simulink model "HOYAS_GRANDES_I"  (R2023b)
settings: Solver=FixedStepDiscrete  StartTime=0.0  StopTime=inf  FixedStep=Ts_Power  RelTol=1e-3  EnableMultiTasking=on
PostLoadFcn:
  | Ts_Power=50e-6;f=50;R_ac=0.12;L_ac=0.08/(2*pi*50);L1=0.17874;L2=0.07596;L3=0.04321;L4=0.01471;L5=0.04751;L6=0.2054;L7=0.17263;L8=0.14418;L9=0.17697;L10=0.19944;L11=0.18905;L12=0.26987;L13=0.1671;L14=0.16874;L15=0.14664;L16=0.12477;L17=0.14989;L18=0.17217;L19=0.19436; load('PV_prof_norm.mat');
InitFcn:
  | Ts_Power=50e-6;f=50;R_ac=0.12;L_ac=0.08/(2*pi*50);L1=0.17874;L2=0.07596;L3=0.04321;L4=0.01471;L5=0.04751;L6=0.2054;L7=0.17263;L8=0.14418;L9=0.17697;L10=0.19944;L11=0.18905;L12=0.26987;L13=0.1671;L14=0.16874;L15=0.14664;L16=0.12477;L17=0.14989;L18=0.17217;L19=0.19436; load('PV_prof_norm.mat');
undefined symbols (not defined in the file or in its folder): D11, Delta, L, X_ac
libraries: spsVoltageMeasurementLib x84, spsCurrentMeasurementLib x75, rtlab x41, spsThreePhaseSeriesRLCBranchLib x38, spsGroundLib x28, powerlib_extras x25, spsThreePhaseDynamicLoadLib x19, eeGeneralControl x4, rteventslib x4, spsThreePhasePISectionLineLib x2, spsThreePhaseTransformerTwoWindingsLib x2, spsPLLLib x1
(part 2 of 4)

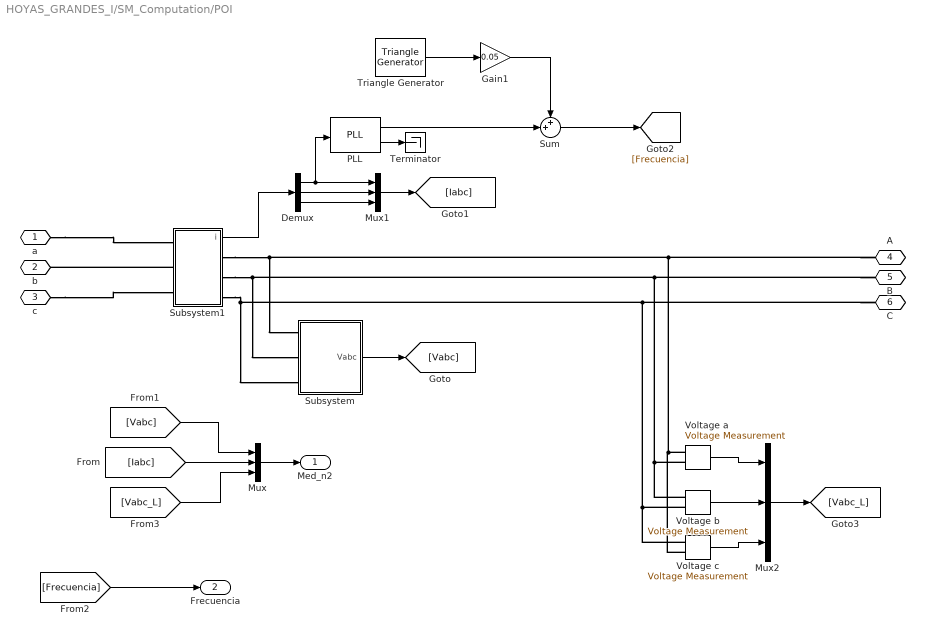
== system HOYAS_GRANDES_I/SM_Computation/POI ==
  Demux : Demux  Outputs=3
  Gain1 : Gain  Gain=0.05
  Mux : Mux  Inputs=3
  Mux1 : Mux  Inputs=3
  Mux2 : Mux  Inputs=3
  PLL : spsPLLLib/PLL  Fmin=45  Par_Init=[0, 50]  ParK=[180, 3200, 1]  TcD=1e-4  MaxRateChangeFreq=12  FilterCutOffFreq=25  Ts=Ts_Power  AGC=on
      settings: LibrarySourceBlock=sps_lib/Control/PLL
  Subsystem : Subsystem
  Subsystem1 : Subsystem
  Sum : Sum  Inputs=++|
  Terminator : Terminator
  Triangle Generator : spsTriangleGeneratorLib/Triangle Generator  Freq=0.1  Phase=0  Ts=Ts_Power
  Voltage a : spsVoltageMeasurementLib/Voltage Measurement  PhasorSimulation=off  OutputType=Complex  PSBequivalent=0
  Voltage b : spsVoltageMeasurementLib/Voltage Measurement  PhasorSimulation=off  OutputType=Complex  PSBequivalent=0
  Voltage c : spsVoltageMeasurementLib/Voltage Measurement  PhasorSimulation=off  OutputType=Complex  PSBequivalent=0
  a : PMIOPort  Side=Right
  b : PMIOPort  Port=2  Side=Right
  c : PMIOPort  Port=3  Side=Right
  A : PMIOPort  Port=4  Side=Left
  B : PMIOPort  Port=5  Side=Left
  C : PMIOPort  Port=6  Side=Left
  Med_n2 : Outport
  Frecuencia : Outport  Port=2
  wires:
  Mux/1 -> Med_n2/1
  [Iabc] -> Mux/2
  [Vabc] -> Mux/1
  Subsystem/1(Vabc) -> [Vabc]
  Mux1/1 -> [Iabc]
  Subsystem1/1(i) -> Demux/1
  Demux/1 -> PLL/1, Mux1/1
  Demux/2 -> Mux1/2
  Demux/3 -> Mux1/3
  PLL/2 -> Terminator/1
  [Frecuencia] -> Frecuencia/1
  Sum/1 -> [Frecuencia]
  Triangle Generator/1 -> Gain1/1
  PLL/1 -> Sum/2
  Gain1/1 -> Sum/1
  Voltage a/1 -> Mux2/1
  Voltage b/1 -> Mux2/2
  Voltage c/1 -> Mux2/3
  Mux2/1 -> [Vabc_L]
  [Vabc_L] -> Mux/3
  connections:
  a/RConn1 -- Subsystem1/LConn1
  Subsystem1/LConn2 -- b/RConn1
  c/RConn1 -- Subsystem1/LConn3
  Voltage c/LConn1 -- Subsystem/LConn3 -- Subsystem1/RConn3 -- C/RConn1 -- Voltage b/LConn2
  Voltage a/LConn1 -- Subsystem/LConn1 -- Subsystem1/RConn1 -- A/RConn1 -- Voltage c/LConn2
  Voltage b/LConn1 -- Subsystem/LConn2 -- Subsystem1/RConn2 -- B/RConn1 -- Voltage a/LConn2

== system HOYAS_GRANDES_I/SM_Computation/Subsystem1 ==
  P_profile : Inport
  P_PPC : Inport  Port=2
  PPC : Constant  Commented=on  Value=0
  Perfil : Constant  Commented=on  Value=3e3
  RTE Conversion : rteventslib/Signal Attributes/RTE Conversion  inputdatatype=RTE Boolean  outputdatatype=Double  compensation=Enabled  nbMaxEvents=10  sampleTime=Ts_Power
      settings: SourceProductName=RT-EVENTS
  RTE Relational Operator1 : rteventslib/Math Operations/RTE Relational Operator  RelationalOperator=>  NumberMaxEvents=1  SampleTime=Ts_Power
      settings: SourceProductName=RT-EVENTS
  Switch : Switch  Criteria=u2 > Threshold  SaturateOnIntegerOverflow=off  InputSameDT=off
  Out1 : Outport
  wires:
  P_profile/1 -> [Perfil]
  P_PPC/1 -> [PPC]
  RTE Relational Operator1/1 -> RTE Conversion/1
  RTE Conversion/1 -> Switch/2
  Switch/1 -> Out1/1
  [Perfil] -> Switch/3, RTE Relational Operator1/1
  [PPC] -> Switch/1, RTE Relational Operator1/2

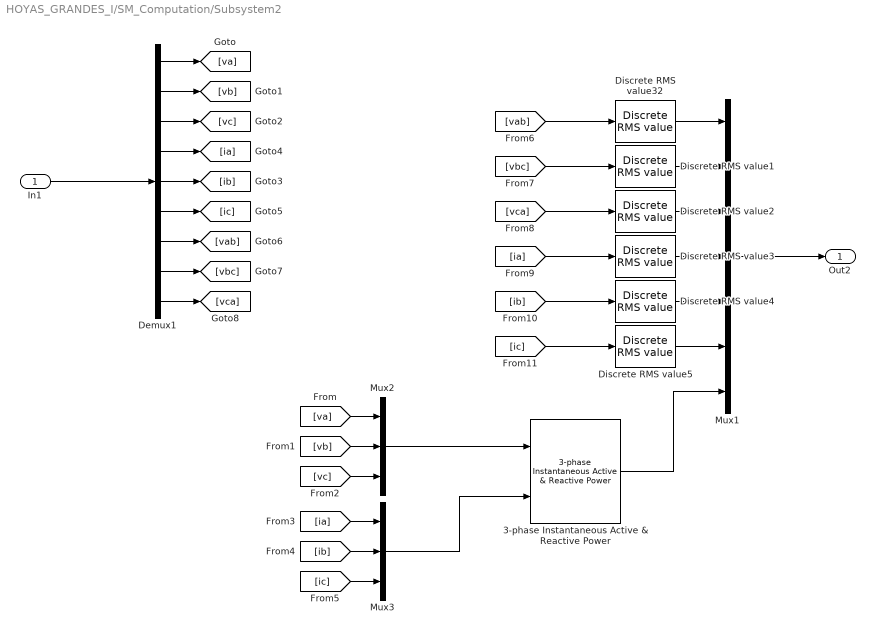
== system HOYAS_GRANDES_I/SM_Computation/Subsystem2 ==
  In1 : Inport
  3-phase Instantaneous Active & Reactive Power : powerlib_extras/Measurements/3-phase  Instantaneous  Active & Reactive Power
  Demux1 : Demux  Outputs=9
  Discrete RMS value1 : powerlib_extras/Discrete Measurements/Discrete  RMS value  Freq=50  Mag_Init=20e3  Ts=Ts_Power
  Discrete RMS value2 : powerlib_extras/Discrete Measurements/Discrete  RMS value  Freq=50  Mag_Init=20e3  Ts=Ts_Power
  Discrete RMS value3 : powerlib_extras/Discrete Measurements/Discrete  RMS value  Freq=50  Mag_Init=0  Ts=Ts_Power
  Discrete RMS value32 : powerlib_extras/Discrete Measurements/Discrete  RMS value  Freq=50  Mag_Init=20e3  Ts=Ts_Power
  Discrete RMS value4 : powerlib_extras/Discrete Measurements/Discrete  RMS value  Freq=50  Mag_Init=0  Ts=Ts_Power
  Discrete RMS value5 : powerlib_extras/Discrete Measurements/Discrete  RMS value  Freq=50  Mag_Init=0  Ts=Ts_Power
  Mux1 : Mux  Inputs=7
  Mux2 : Mux  Inputs=3
  Mux3 : Mux  Inputs=3
  Out2 : Outport
  wires:
  Discrete RMS value5/1 -> Mux1/6
  Discrete RMS value4/1 -> Mux1/5
  Discrete RMS value3/1 -> Mux1/4
  [ic] -> Discrete RMS value5/1
  [ib] -> Discrete RMS value4/1
  [ia] -> Discrete RMS value3/1
  3-phase Instantaneous Active & Reactive Power/1 -> Mux1/7
  [vca] -> Discrete RMS value2/1
  Discrete RMS value2/1 -> Mux1/3
  [vbc] -> Discrete RMS value1/1
  [vab] -> Discrete RMS value32/1
  Demux1/9 -> [vca]
  Demux1/8 -> [vbc]
  Demux1/7 -> [vab]
  [ic] -> Mux3/3
  [ib] -> Mux3/2
  [ia] -> Mux3/1
  [vc] -> Mux2/3
  [vb] -> Mux2/2
  [va] -> Mux2/1
  Mux3/1 -> 3-phase Instantaneous Active & Reactive Power/2
  Mux2/1 -> 3-phase Instantaneous Active & Reactive Power/1
  Demux1/6 -> [ic]
  Demux1/5 -> [ib]
  Demux1/3 -> [vc]
  Demux1/2 -> [vb]
  In1/1 -> Demux1/1
  Demux1/1 -> [va]
  Demux1/4 -> [ia]
  Mux1/1 -> Out2/1
  Discrete RMS value32/1 -> Mux1/1
  Discrete RMS value1/1 -> Mux1/2

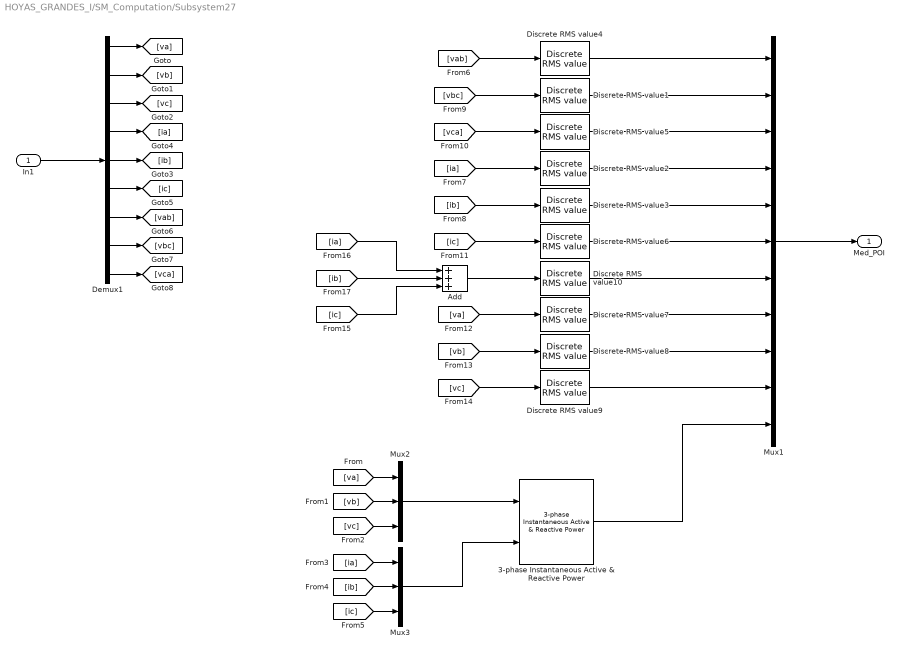
== system HOYAS_GRANDES_I/SM_Computation/Subsystem27 ==
  In1 : Inport
  3-phase Instantaneous Active & Reactive Power : powerlib_extras/Measurements/3-phase  Instantaneous  Active & Reactive Power
  Add : Sum  Inputs=+++
  Demux1 : Demux  Outputs=9
  Discrete RMS value1 : powerlib_extras/Discrete Measurements/Discrete  RMS value  Freq=50  Mag_Init=20e3  Ts=Ts_Power
  Discrete RMS value{2..3,6,10} (4 alike) : powerlib_extras/Discrete Measurements/Discrete  RMS value  Freq=50  Mag_Init=0  Ts=Ts_Power
  Discrete RMS value4 : powerlib_extras/Discrete Measurements/Discrete  RMS value  Freq=50  Mag_Init=20e3  Ts=Ts_Power
  Discrete RMS value5 : powerlib_extras/Discrete Measurements/Discrete  RMS value  Freq=50  Mag_Init=20e3  Ts=Ts_Power
  Discrete RMS value7 : powerlib_extras/Discrete Measurements/Discrete  RMS value  Freq=50  Mag_Init=20e3/sqrt(3)  Ts=Ts_Power
  Discrete RMS value8 : powerlib_extras/Discrete Measurements/Discrete  RMS value  Freq=50  Mag_Init=20e3/sqrt(3)  Ts=Ts_Power
  Discrete RMS value9 : powerlib_extras/Discrete Measurements/Discrete  RMS value  Freq=50  Mag_Init=20e3/sqrt(3)  Ts=Ts_Power
  Mux1 : Mux  Inputs=11
  Mux2 : Mux  Inputs=3
  Mux3 : Mux  Inputs=3
  Med_POI : Outport
  wires:
  [ic] -> Mux3/3
  [ib] -> Mux3/2
  [ia] -> Mux3/1
  [vc] -> Mux2/3
  [vb] -> Mux2/2
  [va] -> Mux2/1
  Mux3/1 -> 3-phase Instantaneous Active & Reactive Power/2
  Mux2/1 -> 3-phase Instantaneous Active & Reactive Power/1
  Demux1/6 -> [ic]
  Demux1/5 -> [ib]
  Demux1/3 -> [vc]
  Demux1/2 -> [vb]
  In1/1 -> Demux1/1
  Demux1/1 -> [va]
  Demux1/4 -> [ia]
  Mux1/1 -> Med_POI/1
  [ia] -> Discrete RMS value2/1
  [ib] -> Discrete RMS value3/1
  Demux1/7 -> [vab]
  Demux1/8 -> [vbc]
  Demux1/9 -> [vca]
  [vab] -> Discrete RMS value4/1
  [vbc] -> Discrete RMS value1/1
  [vca] -> Discrete RMS value5/1
  [ic] -> Discrete RMS value6/1
  [va] -> Discrete RMS value7/1
  [vb] -> Discrete RMS value8/1
  [vc] -> Discrete RMS value9/1
  Discrete RMS value4/1 -> Mux1/1
  Discrete RMS value1/1 -> Mux1/2
  Discrete RMS value5/1 -> Mux1/3
  Discrete RMS value2/1 -> Mux1/4
  Discrete RMS value3/1 -> Mux1/5
  Discrete RMS value6/1 -> Mux1/6
  3-phase Instantaneous Active & Reactive Power/1 -> Mux1/11
  Discrete RMS value9/1 -> Mux1/10
  Discrete RMS value8/1 -> Mux1/9
  Discrete RMS value7/1 -> Mux1/8
  [ic] -> Add/3
  [ib] -> Add/2
  [ia] -> Add/1
  Add/1 -> Discrete RMS value10/1
  Discrete RMS value10/1 -> Mux1/7

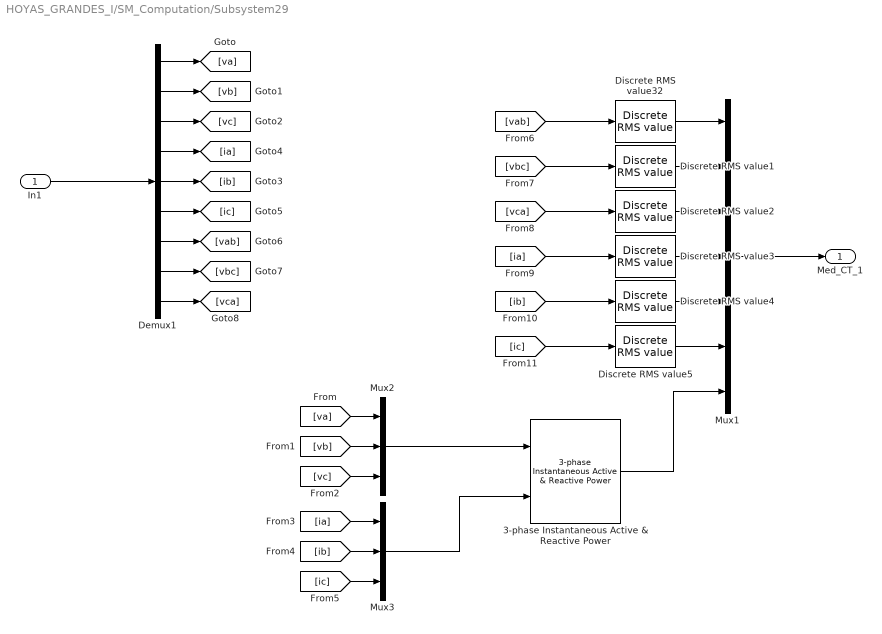
== system HOYAS_GRANDES_I/SM_Computation/Subsystem29 ==
  In1 : Inport
  3-phase Instantaneous Active & Reactive Power : powerlib_extras/Measurements/3-phase  Instantaneous  Active & Reactive Power
  Demux1 : Demux  Outputs=9
  Discrete RMS value1 : powerlib_extras/Discrete Measurements/Discrete  RMS value  Freq=50  Mag_Init=20e3  Ts=Ts_Power
  Discrete RMS value2 : powerlib_extras/Discrete Measurements/Discrete  RMS value  Freq=50  Mag_Init=20e3  Ts=Ts_Power
  Discrete RMS value3 : powerlib_extras/Discrete Measurements/Discrete  RMS value  Freq=50  Mag_Init=0  Ts=Ts_Power
  Discrete RMS value32 : powerlib_extras/Discrete Measurements/Discrete  RMS value  Freq=50  Mag_Init=20e3  Ts=Ts_Power
  Discrete RMS value4 : powerlib_extras/Discrete Measurements/Discrete  RMS value  Freq=50  Mag_Init=0  Ts=Ts_Power
  Discrete RMS value5 : powerlib_extras/Discrete Measurements/Discrete  RMS value  Freq=50  Mag_Init=0  Ts=Ts_Power
  Mux1 : Mux  Inputs=7
  Mux2 : Mux  Inputs=3
  Mux3 : Mux  Inputs=3
  Med_CT_1 : Outport
  wires:
  Discrete RMS value1/1 -> Mux1/2
  Discrete RMS value32/1 -> Mux1/1
  Mux1/1 -> Med_CT_1/1
  Demux1/4 -> [ia]
  Demux1/1 -> [va]
  In1/1 -> Demux1/1
  Demux1/2 -> [vb]
  Demux1/3 -> [vc]
  Demux1/5 -> [ib]
  Demux1/6 -> [ic]
  Mux2/1 -> 3-phase Instantaneous Active & Reactive Power/1
  Mux3/1 -> 3-phase Instantaneous Active & Reactive Power/2
  [va] -> Mux2/1
  [vb] -> Mux2/2
  [vc] -> Mux2/3
  [ia] -> Mux3/1
  [ib] -> Mux3/2
  [ic] -> Mux3/3
  Demux1/7 -> [vab]
  Demux1/8 -> [vbc]
  Demux1/9 -> [vca]
  [vab] -> Discrete RMS value32/1
  [vbc] -> Discrete RMS value1/1
  Discrete RMS value2/1 -> Mux1/3
  [vca] -> Discrete RMS value2/1
  3-phase Instantaneous Active & Reactive Power/1 -> Mux1/7
  [ia] -> Discrete RMS value3/1
  [ib] -> Discrete RMS value4/1
  [ic] -> Discrete RMS value5/1
  Discrete RMS value3/1 -> Mux1/4
  Discrete RMS value4/1 -> Mux1/5
  Discrete RMS value5/1 -> Mux1/6

== system HOYAS_GRANDES_I/SM_Computation/Subsystem31 ==
  P_profile : Inport
  P_PPC : Inport  Port=2
  Constant : Constant
  Multiport Switch3 : MultiPortSwitch  Inputs=2  SaturateOnIntegerOverflow=off  InputSameDT=off
  P_PPC1 : InportShadow  Port=2
  P_profile1 : InportShadow
  RTE Conversion : rteventslib/Signal Attributes/RTE Conversion  inputdatatype=RTE Boolean  outputdatatype=Double  compensation=Enabled  nbMaxEvents=10  sampleTime=Ts_Power
      settings: SourceProductName=RT-EVENTS
  RTE Relational Operator : rteventslib/Math Operations/RTE Relational Operator  RelationalOperator=>=  NumberMaxEvents=1  SampleTime=Ts_Power
      settings: SourceProductName=RT-EVENTS
  Sum2 : Sum  Inputs=|++
  Out1 : Outport
  wires:
  P_profile/1 -> RTE Relational Operator/2
  P_PPC/1 -> RTE Relational Operator/1
  RTE Conversion/1 -> Sum2/1
  Sum2/1 -> Multiport Switch3/1
  Constant/1 -> Sum2/2
  P_PPC1/1 -> Multiport Switch3/3
  P_profile1/1 -> Multiport Switch3/2
  RTE Relational Operator/1 -> RTE Conversion/1
  Multiport Switch3/1 -> Out1/1

== system HOYAS_GRANDES_I/SM_Computation/save ==
  meas_tratadas : Inport
  OpWriteFile1 : rtlab/DataLogging/OpWriteFile  Static_File=on  varname=opvar  Filename=myfile.mat  rtpath='./'  nrtpath='.\'  Acq_Group=26  file_size=100000000  write_offline=off  Sim_Mode=off  Nb_Samples=144  Buffer_size=1000000
      settings: SourceProductName=RT-LAB  Decimation=1/100e-5
  Out1 : Outport
  Out2 : Outport  Port=2
  wires:
  OpWriteFile1/1 -> Out1/1
  OpWriteFile1/2 -> Out2/1
  meas_tratadas/1 -> OpWriteFile1/1

== system HOYAS_GRANDES_I/SM_Computation/HG1_CT.01-CT.02-LMT.1/Subsystem ==
  Ground2 : spsGroundLib/Ground  LConnTagsString=a
  Mux1 : Mux  Inputs=3
  Voltage a : spsVoltageMeasurementLib/Voltage Measurement  PhasorSimulation=off  OutputType=Complex  PSBequivalent=0
  Voltage b : spsVoltageMeasurementLib/Voltage Measurement  PhasorSimulation=off  OutputType=Complex  PSBequivalent=0
  Voltage c : spsVoltageMeasurementLib/Voltage Measurement  PhasorSimulation=off  OutputType=Complex  PSBequivalent=0
  Va : PMIOPort  Side=Left
  Vb : PMIOPort  Port=2  Side=Left
  Vc : PMIOPort  Port=3  Side=Left
  Vabc : Outport
  wires:
  Voltage c/1 -> Mux1/3
  Voltage a/1 -> Mux1/1
  Mux1/1 -> Vabc/1
  Voltage b/1 -> Mux1/2
  connections:
  Voltage c/LConn1 -- Vc/RConn1
  Voltage a/LConn1 -- Va/RConn1
  Voltage a/LConn2 -- Voltage b/LConn2 -- Voltage c/LConn2 -- Ground2/LConn1
  Voltage b/LConn1 -- Vb/RConn1

== system HOYAS_GRANDES_I/SM_Computation/HG1_CT.01-CT.02-LMT.1/Subsystem1 ==
  Current Measurement : spsCurrentMeasurementLib/Current Measurement  PhasorSimulation=off  OutputType=Complex  PSBequivalent=0
  Current Measurement1 : spsCurrentMeasurementLib/Current Measurement  PhasorSimulation=off  OutputType=Complex  PSBequivalent=0
  Current Measurement2 : spsCurrentMeasurementLib/Current Measurement  PhasorSimulation=off  OutputType=Complex  PSBequivalent=0
  Mux : Mux  Inputs=3
  a : PMIOPort  Side=Right
  ia : PMIOPort  Port=2  Side=Left
  ib : PMIOPort  Port=3  Side=Left
  b : PMIOPort  Port=4  Side=Right
  ic : PMIOPort  Port=5  Side=Left
  c : PMIOPort  Port=6  Side=Right
  i : Outport
  wires:
  Current Measurement1/1 -> Mux/2
  Current Measurement2/1 -> Mux/3
  Current Measurement/1 -> Mux/1
  Mux/1 -> i/1
  connections:
  ic/RConn1 -- Current Measurement2/LConn1
  ia/RConn1 -- Current Measurement/LConn1
  Current Measurement1/LConn1 -- ib/RConn1
  Current Measurement2/RConn1 -- c/RConn1
  Current Measurement/RConn1 -- a/RConn1
  Current Measurement1/RConn1 -- b/RConn1

== system HOYAS_GRANDES_I/SM_Computation/HG1_CT.01-CT.02-LMT.2/Subsystem ==
  Ground2 : spsGroundLib/Ground  LConnTagsString=a
  Mux1 : Mux  Inputs=3
  Voltage a : spsVoltageMeasurementLib/Voltage Measurement  PhasorSimulation=off  OutputType=Complex  PSBequivalent=0
  Voltage b : spsVoltageMeasurementLib/Voltage Measurement  PhasorSimulation=off  OutputType=Complex  PSBequivalent=0
  Voltage c : spsVoltageMeasurementLib/Voltage Measurement  PhasorSimulation=off  OutputType=Complex  PSBequivalent=0
  Va : PMIOPort  Side=Left
  Vb : PMIOPort  Port=2  Side=Left
  Vc : PMIOPort  Port=3  Side=Left
  Vabc : Outport
  wires:
  Voltage b/1 -> Mux1/2
  Mux1/1 -> Vabc/1
  Voltage a/1 -> Mux1/1
  Voltage c/1 -> Mux1/3
  connections:
  Voltage b/LConn1 -- Vb/RConn1
  Ground2/LConn1 -- Voltage c/LConn2 -- Voltage b/LConn2 -- Voltage a/LConn2
  Voltage a/LConn1 -- Va/RConn1
  Voltage c/LConn1 -- Vc/RConn1

== system HOYAS_GRANDES_I/SM_Computation/HG1_CT.01-CT.02-LMT.2/Subsystem1 ==
  Current Measurement : spsCurrentMeasurementLib/Current Measurement  PhasorSimulation=off  OutputType=Complex  PSBequivalent=0
  Current Measurement1 : spsCurrentMeasurementLib/Current Measurement  PhasorSimulation=off  OutputType=Complex  PSBequivalent=0
  Current Measurement2 : spsCurrentMeasurementLib/Current Measurement  PhasorSimulation=off  OutputType=Complex  PSBequivalent=0
  Mux : Mux  Inputs=3
  a : PMIOPort  Side=Right
  ia : PMIOPort  Port=2  Side=Left
  ib : PMIOPort  Port=3  Side=Left
  b : PMIOPort  Port=4  Side=Right
  ic : PMIOPort  Port=5  Side=Left
  c : PMIOPort  Port=6  Side=Right
  i : Outport
  wires:
  Mux/1 -> i/1
  Current Measurement/1 -> Mux/1
  Current Measurement2/1 -> Mux/3
  Current Measurement1/1 -> Mux/2
  connections:
  Current Measurement1/RConn1 -- b/RConn1
  Current Measurement/RConn1 -- a/RConn1
  Current Measurement2/RConn1 -- c/RConn1
  Current Measurement1/LConn1 -- ib/RConn1
  ia/RConn1 -- Current Measurement/LConn1
  ic/RConn1 -- Current Measurement2/LConn1

== system HOYAS_GRANDES_I/SM_Computation/HG1_CT.02-CS-LMT.2/Subsystem ==
  Ground2 : spsGroundLib/Ground  LConnTagsString=a
  Mux1 : Mux  Inputs=3
  Voltage a : spsVoltageMeasurementLib/Voltage Measurement  PhasorSimulation=off  OutputType=Complex  PSBequivalent=0
  Voltage b : spsVoltageMeasurementLib/Voltage Measurement  PhasorSimulation=off  OutputType=Complex  PSBequivalent=0
  Voltage c : spsVoltageMeasurementLib/Voltage Measurement  PhasorSimulation=off  OutputType=Complex  PSBequivalent=0
  Va : PMIOPort  Side=Left
  Vb : PMIOPort  Port=2  Side=Left
  Vc : PMIOPort  Port=3  Side=Left
  Vabc : Outport
  wires:
  Voltage b/1 -> Mux1/2
  Mux1/1 -> Vabc/1
  Voltage a/1 -> Mux1/1
  Voltage c/1 -> Mux1/3
  connections:
  Voltage b/LConn1 -- Vb/RConn1
  Ground2/LConn1 -- Voltage c/LConn2 -- Voltage b/LConn2 -- Voltage a/LConn2
  Voltage a/LConn1 -- Va/RConn1
  Voltage c/LConn1 -- Vc/RConn1

== system HOYAS_GRANDES_I/SM_Computation/HG1_CT.02-CS-LMT.2/Subsystem1 ==
  Current Measurement : spsCurrentMeasurementLib/Current Measurement  PhasorSimulation=off  OutputType=Complex  PSBequivalent=0
  Current Measurement1 : spsCurrentMeasurementLib/Current Measurement  PhasorSimulation=off  OutputType=Complex  PSBequivalent=0
  Current Measurement2 : spsCurrentMeasurementLib/Current Measurement  PhasorSimulation=off  OutputType=Complex  PSBequivalent=0
  Mux : Mux  Inputs=3
  a : PMIOPort  Side=Right
  ia : PMIOPort  Port=2  Side=Left
  ib : PMIOPort  Port=3  Side=Left
  b : PMIOPort  Port=4  Side=Right
  ic : PMIOPort  Port=5  Side=Left
  c : PMIOPort  Port=6  Side=Right
  i : Outport
  wires:
  Current Measurement1/1 -> Mux/2
  Current Measurement2/1 -> Mux/3
  Current Measurement/1 -> Mux/1
  Mux/1 -> i/1
  connections:
  ic/RConn1 -- Current Measurement2/LConn1
  ia/RConn1 -- Current Measurement/LConn1
  Current Measurement1/LConn1 -- ib/RConn1
  Current Measurement2/RConn1 -- c/RConn1
  Current Measurement/RConn1 -- a/RConn1
  Current Measurement1/RConn1 -- b/RConn1

== system HOYAS_GRANDES_I/SM_Computation/HOYAS GRANDES CT01/HG.1-CT.1-INV.01 ==
  PQ : Inport
  Three-Phase Dynamic Load : spsThreePhaseDynamicLoadLib/Three-Phase Dynamic Load  NominalVoltage=[ 800 50 ]  ActiveReactivePowers=[0 0]  PositiveSequence=[1 0]  ExternalControl=on  NpNq=[1.3 2]  TimeConstants="[0  0  0  0]"  MinimumVoltage=0.7  Tfilter=1e-4  LoadFlowParameters=[4,0,0,0,0]
      settings: LibrarySourceBlock=|
      | sps_lib/Passives/Three-Phase
      | Dynamic Load
  Three-Phase Series RLC Branch10 : spsThreePhaseSeriesRLCBranchLib/Three-Phase Series RLC Branch  LConnTagsString=A|B|C  RConnTagsString=A|B|C  BranchType=R  Resistance=1e6  Inductance=X_ac*L  Capacitance=1e-6  Measurements=None
  A : PMIOPort  Side=Right
  B : PMIOPort  Port=2  Side=Right
  C : PMIOPort  Port=3  Side=Right
  m : Outport
  wires:
  Three-Phase Dynamic Load/1 -> m/1
  PQ/1 -> Three-Phase Dynamic Load/1
  connections:
  Three-Phase Dynamic Load/LConn3 -- C/RConn1 -- Three-Phase Series RLC Branch10/RConn3
  Three-Phase Dynamic Load/LConn2 -- Three-Phase Series RLC Branch10/RConn2 -- B/RConn1
  Three-Phase Series RLC Branch10/LConn1 -- Three-Phase Series RLC Branch10/LConn3 -- Three-Phase Series RLC Branch10/LConn2
  Three-Phase Series RLC Branch10/RConn1 -- Three-Phase Dynamic Load/LConn1 -- A/RConn1

== system HOYAS_GRANDES_I/SM_Computation/HOYAS GRANDES CT01/HG.1-CT.1-INV.02 ==
  PQ : Inport
  Three-Phase Dynamic Load : spsThreePhaseDynamicLoadLib/Three-Phase Dynamic Load  NominalVoltage=[ 800 50 ]  ActiveReactivePowers=[0 0]  PositiveSequence=[1 0]  ExternalControl=on  NpNq=[1.3 2]  TimeConstants="[0  0  0  0]"  MinimumVoltage=0.7  Tfilter=1e-4  LoadFlowParameters=[4,0,0,0,0]
      settings: LibrarySourceBlock=|
      | sps_lib/Passives/Three-Phase
      | Dynamic Load
  Three-Phase Series RLC Branch10 : spsThreePhaseSeriesRLCBranchLib/Three-Phase Series RLC Branch  LConnTagsString=A|B|C  RConnTagsString=A|B|C  BranchType=R  Resistance=1e6  Inductance=X_ac*L  Capacitance=1e-6  Measurements=None
  A : PMIOPort  Side=Right
  B : PMIOPort  Port=2  Side=Right
  C : PMIOPort  Port=3  Side=Right
  m : Outport
  wires:
  PQ/1 -> Three-Phase Dynamic Load/1
  Three-Phase Dynamic Load/1 -> m/1
  connections:
  Three-Phase Dynamic Load/LConn1 -- Three-Phase Series RLC Branch10/RConn1 -- A/RConn1
  Three-Phase Series RLC Branch10/LConn3 -- Three-Phase Series RLC Branch10/LConn1 -- Three-Phase Series RLC Branch10/LConn2
  B/RConn1 -- Three-Phase Series RLC Branch10/RConn2 -- Three-Phase Dynamic Load/LConn2
  C/RConn1 -- Three-Phase Dynamic Load/LConn3 -- Three-Phase Series RLC Branch10/RConn3

== system HOYAS_GRANDES_I/SM_Computation/HOYAS GRANDES CT01/HG.1-CT.1-INV.03 ==
  PQ : Inport
  Three-Phase Dynamic Load : spsThreePhaseDynamicLoadLib/Three-Phase Dynamic Load  NominalVoltage=[ 800 50 ]  ActiveReactivePowers=[0 0]  PositiveSequence=[1 0]  ExternalControl=on  NpNq=[1.3 2]  TimeConstants="[0  0  0  0]"  MinimumVoltage=0.7  Tfilter=1e-4  LoadFlowParameters=[4,0,0,0,0]
      settings: LibrarySourceBlock=|
      | sps_lib/Passives/Three-Phase
      | Dynamic Load
  Three-Phase Series RLC Branch10 : spsThreePhaseSeriesRLCBranchLib/Three-Phase Series RLC Branch  LConnTagsString=A|B|C  RConnTagsString=A|B|C  BranchType=R  Resistance=1e6  Inductance=X_ac*L  Capacitance=1e-6  Measurements=None
  A : PMIOPort  Side=Right
  B : PMIOPort  Port=2  Side=Right
  C : PMIOPort  Port=3  Side=Right
  m : Outport
  wires:
  Three-Phase Dynamic Load/1 -> m/1
  PQ/1 -> Three-Phase Dynamic Load/1
  connections:
  Three-Phase Series RLC Branch10/RConn3 -- Three-Phase Dynamic Load/LConn3 -- C/RConn1
  Three-Phase Dynamic Load/LConn2 -- Three-Phase Series RLC Branch10/RConn2 -- B/RConn1
  Three-Phase Series RLC Branch10/LConn2 -- Three-Phase Series RLC Branch10/LConn1 -- Three-Phase Series RLC Branch10/LConn3
  A/RConn1 -- Three-Phase Series RLC Branch10/RConn1 -- Three-Phase Dynamic Load/LConn1

== system HOYAS_GRANDES_I/SM_Computation/HOYAS GRANDES CT01/HG.1-CT.1-INV.04 ==
  PQ : Inport
  Three-Phase Dynamic Load : spsThreePhaseDynamicLoadLib/Three-Phase Dynamic Load  NominalVoltage=[ 800 50 ]  ActiveReactivePowers=[0 0]  PositiveSequence=[1 0]  ExternalControl=on  NpNq=[1.3 2]  TimeConstants="[0  0  0  0]"  MinimumVoltage=0.7  Tfilter=1e-4  LoadFlowParameters=[4,0,0,0,0]
      settings: LibrarySourceBlock=|
      | sps_lib/Passives/Three-Phase
      | Dynamic Load
  Three-Phase Series RLC Branch10 : spsThreePhaseSeriesRLCBranchLib/Three-Phase Series RLC Branch  LConnTagsString=A|B|C  RConnTagsString=A|B|C  BranchType=R  Resistance=1e6  Inductance=X_ac*L  Capacitance=1e-6  Measurements=None
  A : PMIOPort  Side=Right
  B : PMIOPort  Port=2  Side=Right
  C : PMIOPort  Port=3  Side=Right
  m : Outport
  wires:
  PQ/1 -> Three-Phase Dynamic Load/1
  Three-Phase Dynamic Load/1 -> m/1
  connections:
  Three-Phase Dynamic Load/LConn1 -- Three-Phase Series RLC Branch10/RConn1 -- A/RConn1
  Three-Phase Series RLC Branch10/LConn3 -- Three-Phase Series RLC Branch10/LConn1 -- Three-Phase Series RLC Branch10/LConn2
  B/RConn1 -- Three-Phase Series RLC Branch10/RConn2 -- Three-Phase Dynamic Load/LConn2
  C/RConn1 -- Three-Phase Dynamic Load/LConn3 -- Three-Phase Series RLC Branch10/RConn3

== system HOYAS_GRANDES_I/SM_Computation/HOYAS GRANDES CT01/HG.1-CT.1-INV.05 ==
  PQ : Inport
  Three-Phase Dynamic Load : spsThreePhaseDynamicLoadLib/Three-Phase Dynamic Load  NominalVoltage=[ 800 50 ]  ActiveReactivePowers=[0 0]  PositiveSequence=[1 0]  ExternalControl=on  NpNq=[1.3 2]  TimeConstants="[0  0  0  0]"  MinimumVoltage=0.7  Tfilter=1e-4  LoadFlowParameters=[4,0,0,0,0]
      settings: LibrarySourceBlock=|
      | sps_lib/Passives/Three-Phase
      | Dynamic Load
  Three-Phase Series RLC Branch10 : spsThreePhaseSeriesRLCBranchLib/Three-Phase Series RLC Branch  LConnTagsString=A|B|C  RConnTagsString=A|B|C  BranchType=R  Resistance=1e6  Inductance=X_ac*L  Capacitance=1e-6  Measurements=None
  A : PMIOPort  Side=Right
  B : PMIOPort  Port=2  Side=Right
  C : PMIOPort  Port=3  Side=Right
  m : Outport
  wires:
  Three-Phase Dynamic Load/1 -> m/1
  PQ/1 -> Three-Phase Dynamic Load/1
  connections:
  Three-Phase Series RLC Branch10/RConn3 -- Three-Phase Dynamic Load/LConn3 -- C/RConn1
  Three-Phase Dynamic Load/LConn2 -- Three-Phase Series RLC Branch10/RConn2 -- B/RConn1
  Three-Phase Series RLC Branch10/LConn2 -- Three-Phase Series RLC Branch10/LConn1 -- Three-Phase Series RLC Branch10/LConn3
  A/RConn1 -- Three-Phase Series RLC Branch10/RConn1 -- Three-Phase Dynamic Load/LConn1

== system HOYAS_GRANDES_I/SM_Computation/HOYAS GRANDES CT01/HG.1-CT.1-INV.06 ==
  PQ : Inport
  Three-Phase Dynamic Load : spsThreePhaseDynamicLoadLib/Three-Phase Dynamic Load  NominalVoltage=[ 800 50 ]  ActiveReactivePowers=[0 0]  PositiveSequence=[1 0]  ExternalControl=on  NpNq=[1.3 2]  TimeConstants="[0  0  0  0]"  MinimumVoltage=0.7  Tfilter=1e-4  LoadFlowParameters=[4,0,0,0,0]
      settings: LibrarySourceBlock=|
      | sps_lib/Passives/Three-Phase
      | Dynamic Load
  Three-Phase Series RLC Branch10 : spsThreePhaseSeriesRLCBranchLib/Three-Phase Series RLC Branch  LConnTagsString=A|B|C  RConnTagsString=A|B|C  BranchType=R  Resistance=1e6  Inductance=X_ac*L  Capacitance=1e-6  Measurements=None
  A : PMIOPort  Side=Right
  B : PMIOPort  Port=2  Side=Right
  C : PMIOPort  Port=3  Side=Right
  m : Outport
  wires:
  PQ/1 -> Three-Phase Dynamic Load/1
  Three-Phase Dynamic Load/1 -> m/1
  connections:
  Three-Phase Dynamic Load/LConn1 -- Three-Phase Series RLC Branch10/RConn1 -- A/RConn1
  Three-Phase Series RLC Branch10/LConn3 -- Three-Phase Series RLC Branch10/LConn1 -- Three-Phase Series RLC Branch10/LConn2
  B/RConn1 -- Three-Phase Series RLC Branch10/RConn2 -- Three-Phase Dynamic Load/LConn2
  C/RConn1 -- Three-Phase Dynamic Load/LConn3 -- Three-Phase Series RLC Branch10/RConn3

== system HOYAS_GRANDES_I/SM_Computation/HOYAS GRANDES CT01/HG.1-CT.1-INV.07 ==
  PQ : Inport
  Three-Phase Dynamic Load : spsThreePhaseDynamicLoadLib/Three-Phase Dynamic Load  NominalVoltage=[ 800 50 ]  ActiveReactivePowers=[0 0]  PositiveSequence=[1 0]  ExternalControl=on  NpNq=[1.3 2]  TimeConstants="[0  0  0  0]"  MinimumVoltage=0.7  Tfilter=1e-4  LoadFlowParameters=[4,0,0,0,0]
      settings: LibrarySourceBlock=|
      | sps_lib/Passives/Three-Phase
      | Dynamic Load
  Three-Phase Series RLC Branch10 : spsThreePhaseSeriesRLCBranchLib/Three-Phase Series RLC Branch  LConnTagsString=A|B|C  RConnTagsString=A|B|C  BranchType=R  Resistance=1e6  Inductance=X_ac*L  Capacitance=1e-6  Measurements=None
  A : PMIOPort  Side=Right
  B : PMIOPort  Port=2  Side=Right
  C : PMIOPort  Port=3  Side=Right
  m : Outport
  wires:
  Three-Phase Dynamic Load/1 -> m/1
  PQ/1 -> Three-Phase Dynamic Load/1
  connections:
  Three-Phase Series RLC Branch10/RConn3 -- Three-Phase Dynamic Load/LConn3 -- C/RConn1
  Three-Phase Dynamic Load/LConn2 -- Three-Phase Series RLC Branch10/RConn2 -- B/RConn1
  Three-Phase Series RLC Branch10/LConn2 -- Three-Phase Series RLC Branch10/LConn1 -- Three-Phase Series RLC Branch10/LConn3
  A/RConn1 -- Three-Phase Series RLC Branch10/RConn1 -- Three-Phase Dynamic Load/LConn1

== system HOYAS_GRANDES_I/SM_Computation/HOYAS GRANDES CT01/HG.1-CT.1-INV.08 ==
  PQ : Inport
  Three-Phase Dynamic Load : spsThreePhaseDynamicLoadLib/Three-Phase Dynamic Load  NominalVoltage=[ 800 50 ]  ActiveReactivePowers=[0 0]  PositiveSequence=[1 0]  ExternalControl=on  NpNq=[1.3 2]  TimeConstants="[0  0  0  0]"  MinimumVoltage=0.7  Tfilter=1e-4  LoadFlowParameters=[4,0,0,0,0]
      settings: LibrarySourceBlock=|
      | sps_lib/Passives/Three-Phase
      | Dynamic Load
  Three-Phase Series RLC Branch10 : spsThreePhaseSeriesRLCBranchLib/Three-Phase Series RLC Branch  LConnTagsString=A|B|C  RConnTagsString=A|B|C  BranchType=R  Resistance=1e6  Inductance=X_ac*L  Capacitance=1e-6  Measurements=None
  A : PMIOPort  Side=Right
  B : PMIOPort  Port=2  Side=Right
  C : PMIOPort  Port=3  Side=Right
  m : Outport
  wires:
  PQ/1 -> Three-Phase Dynamic Load/1
  Three-Phase Dynamic Load/1 -> m/1
  connections:
  Three-Phase Dynamic Load/LConn1 -- Three-Phase Series RLC Branch10/RConn1 -- A/RConn1
  Three-Phase Series RLC Branch10/LConn3 -- Three-Phase Series RLC Branch10/LConn1 -- Three-Phase Series RLC Branch10/LConn2
  B/RConn1 -- Three-Phase Series RLC Branch10/RConn2 -- Three-Phase Dynamic Load/LConn2
  C/RConn1 -- Three-Phase Dynamic Load/LConn3 -- Three-Phase Series RLC Branch10/RConn3

== system HOYAS_GRANDES_I/SM_Computation/HOYAS GRANDES CT01/HG.1-CT.1-INV.09 ==
  PQ : Inport
  Three-Phase Dynamic Load : spsThreePhaseDynamicLoadLib/Three-Phase Dynamic Load  NominalVoltage=[ 800 50 ]  ActiveReactivePowers=[0 0]  PositiveSequence=[1 0]  ExternalControl=on  NpNq=[1.3 2]  TimeConstants="[0  0  0  0]"  MinimumVoltage=0.7  Tfilter=1e-4  LoadFlowParameters=[4,0,0,0,0]
      settings: LibrarySourceBlock=|
      | sps_lib/Passives/Three-Phase
      | Dynamic Load
  Three-Phase Series RLC Branch10 : spsThreePhaseSeriesRLCBranchLib/Three-Phase Series RLC Branch  LConnTagsString=A|B|C  RConnTagsString=A|B|C  BranchType=R  Resistance=1e6  Inductance=X_ac*L  Capacitance=1e-6  Measurements=None
  A : PMIOPort  Side=Right
  B : PMIOPort  Port=2  Side=Right
  C : PMIOPort  Port=3  Side=Right
  m : Outport
  wires:
  Three-Phase Dynamic Load/1 -> m/1
  PQ/1 -> Three-Phase Dynamic Load/1
  connections:
  Three-Phase Series RLC Branch10/RConn3 -- Three-Phase Dynamic Load/LConn3 -- C/RConn1
  Three-Phase Dynamic Load/LConn2 -- Three-Phase Series RLC Branch10/RConn2 -- B/RConn1
  Three-Phase Series RLC Branch10/LConn2 -- Three-Phase Series RLC Branch10/LConn1 -- Three-Phase Series RLC Branch10/LConn3
  A/RConn1 -- Three-Phase Series RLC Branch10/RConn1 -- Three-Phase Dynamic Load/LConn1

== system HOYAS_GRANDES_I/SM_Computation/HOYAS GRANDES CT01/HG.1-CT.1-INV.10 ==
  PQ : Inport
  Three-Phase Dynamic Load : spsThreePhaseDynamicLoadLib/Three-Phase Dynamic Load  NominalVoltage=[ 800 50 ]  ActiveReactivePowers=[0 0]  PositiveSequence=[1 0]  ExternalControl=on  NpNq=[1.3 2]  TimeConstants="[0  0  0  0]"  MinimumVoltage=0.7  Tfilter=1e-4  LoadFlowParameters=[4,0,0,0,0]
      settings: LibrarySourceBlock=|
      | sps_lib/Passives/Three-Phase
      | Dynamic Load
  Three-Phase Series RLC Branch10 : spsThreePhaseSeriesRLCBranchLib/Three-Phase Series RLC Branch  LConnTagsString=A|B|C  RConnTagsString=A|B|C  BranchType=R  Resistance=1e6  Inductance=X_ac*L  Capacitance=1e-6  Measurements=None
  A : PMIOPort  Side=Right
  B : PMIOPort  Port=2  Side=Right
  C : PMIOPort  Port=3  Side=Right
  m : Outport
  wires:
  PQ/1 -> Three-Phase Dynamic Load/1
  Three-Phase Dynamic Load/1 -> m/1
  connections:
  Three-Phase Dynamic Load/LConn1 -- Three-Phase Series RLC Branch10/RConn1 -- A/RConn1
  Three-Phase Series RLC Branch10/LConn3 -- Three-Phase Series RLC Branch10/LConn1 -- Three-Phase Series RLC Branch10/LConn2
  B/RConn1 -- Three-Phase Series RLC Branch10/RConn2 -- Three-Phase Dynamic Load/LConn2
  C/RConn1 -- Three-Phase Dynamic Load/LConn3 -- Three-Phase Series RLC Branch10/RConn3

== system HOYAS_GRANDES_I/SM_Computation/HOYAS GRANDES CT01/HG.1_CT.1-INV.01 ==
  Mux : Mux  Inputs=2
  Subsystem : Subsystem
  Subsystem1 : Subsystem
  a : PMIOPort  Side=Right
  b : PMIOPort  Port=2  Side=Right
  c : PMIOPort  Port=3  Side=Right
  A : PMIOPort  Port=4  Side=Left
  B : PMIOPort  Port=5  Side=Left
  C : PMIOPort  Port=6  Side=Left
  Med_n2 : Outport
  wires:
  Subsystem/1(Vabc) -> [Vabc]
  Subsystem1/1(i) -> [Iabc]
  [Vabc] -> Mux/1
  [Iabc] -> Mux/2
  Mux/1 -> Med_n2/1
  connections:
  Subsystem1/RConn2 -- B/RConn1 -- Subsystem/LConn2
  Subsystem1/RConn1 -- A/RConn1 -- Subsystem/LConn1
  Subsystem1/RConn3 -- C/RConn1 -- Subsystem/LConn3
  c/RConn1 -- Subsystem1/LConn3
  Subsystem1/LConn2 -- b/RConn1
  a/RConn1 -- Subsystem1/LConn1

== system HOYAS_GRANDES_I/SM_Computation/HOYAS GRANDES CT01/HG.1_CT.1-INV.02 ==
  Mux : Mux  Inputs=2
  Subsystem : Subsystem
  Subsystem1 : Subsystem
  a : PMIOPort  Side=Right
  b : PMIOPort  Port=2  Side=Right
  c : PMIOPort  Port=3  Side=Right
  A : PMIOPort  Port=4  Side=Left
  B : PMIOPort  Port=5  Side=Left
  C : PMIOPort  Port=6  Side=Left
  Med_n2 : Outport
  wires:
  Mux/1 -> Med_n2/1
  [Iabc] -> Mux/2
  [Vabc] -> Mux/1
  Subsystem1/1(i) -> [Iabc]
  Subsystem/1(Vabc) -> [Vabc]
  connections:
  a/RConn1 -- Subsystem1/LConn1
  Subsystem1/LConn2 -- b/RConn1
  c/RConn1 -- Subsystem1/LConn3
  C/RConn1 -- Subsystem1/RConn3 -- Subsystem/LConn3
  A/RConn1 -- Subsystem/LConn1 -- Subsystem1/RConn1
  B/RConn1 -- Subsystem1/RConn2 -- Subsystem/LConn2

== system HOYAS_GRANDES_I/SM_Computation/HOYAS GRANDES CT01/HG.1_CT.1-INV.03 ==
  Mux : Mux  Inputs=2
  Subsystem : Subsystem
  Subsystem1 : Subsystem
  a : PMIOPort  Side=Right
  b : PMIOPort  Port=2  Side=Right
  c : PMIOPort  Port=3  Side=Right
  A : PMIOPort  Port=4  Side=Left
  B : PMIOPort  Port=5  Side=Left
  C : PMIOPort  Port=6  Side=Left
  Med_n2 : Outport
  wires:
  Subsystem/1(Vabc) -> [Vabc]
  Subsystem1/1(i) -> [Iabc]
  [Vabc] -> Mux/1
  [Iabc] -> Mux/2
  Mux/1 -> Med_n2/1
  connections:
  Subsystem/LConn2 -- Subsystem1/RConn2 -- B/RConn1
  Subsystem1/RConn1 -- Subsystem/LConn1 -- A/RConn1
  Subsystem/LConn3 -- Subsystem1/RConn3 -- C/RConn1
  c/RConn1 -- Subsystem1/LConn3
  Subsystem1/LConn2 -- b/RConn1
  a/RConn1 -- Subsystem1/LConn1

== system HOYAS_GRANDES_I/SM_Computation/HOYAS GRANDES CT01/HG.1_CT.1-INV.04 ==
  Mux : Mux  Inputs=2
  Subsystem : Subsystem
  Subsystem1 : Subsystem
  a : PMIOPort  Side=Right
  b : PMIOPort  Port=2  Side=Right
  c : PMIOPort  Port=3  Side=Right
  A : PMIOPort  Port=4  Side=Left
  B : PMIOPort  Port=5  Side=Left
  C : PMIOPort  Port=6  Side=Left
  Med_n2 : Outport
  wires:
  Mux/1 -> Med_n2/1
  [Iabc] -> Mux/2
  [Vabc] -> Mux/1
  Subsystem1/1(i) -> [Iabc]
  Subsystem/1(Vabc) -> [Vabc]
  connections:
  a/RConn1 -- Subsystem1/LConn1
  Subsystem1/LConn2 -- b/RConn1
  c/RConn1 -- Subsystem1/LConn3
  C/RConn1 -- Subsystem1/RConn3 -- Subsystem/LConn3
  A/RConn1 -- Subsystem/LConn1 -- Subsystem1/RConn1
  B/RConn1 -- Subsystem1/RConn2 -- Subsystem/LConn2

== system HOYAS_GRANDES_I/SM_Computation/HOYAS GRANDES CT01/HG.1_CT.1-INV.05 ==
  Mux : Mux  Inputs=2
  Subsystem : Subsystem
  Subsystem1 : Subsystem
  a : PMIOPort  Side=Right
  b : PMIOPort  Port=2  Side=Right
  c : PMIOPort  Port=3  Side=Right
  A : PMIOPort  Port=4  Side=Left
  B : PMIOPort  Port=5  Side=Left
  C : PMIOPort  Port=6  Side=Left
  Med_n2 : Outport
  wires:
  Subsystem/1(Vabc) -> [Vabc]
  Subsystem1/1(i) -> [Iabc]
  [Vabc] -> Mux/1
  [Iabc] -> Mux/2
  Mux/1 -> Med_n2/1
  connections:
  Subsystem/LConn2 -- Subsystem1/RConn2 -- B/RConn1
  Subsystem1/RConn1 -- Subsystem/LConn1 -- A/RConn1
  Subsystem/LConn3 -- Subsystem1/RConn3 -- C/RConn1
  c/RConn1 -- Subsystem1/LConn3
  Subsystem1/LConn2 -- b/RConn1
  a/RConn1 -- Subsystem1/LConn1

== system HOYAS_GRANDES_I/SM_Computation/HOYAS GRANDES CT01/HG.1_CT.1-INV.06 ==
  Mux : Mux  Inputs=2
  Subsystem : Subsystem
  Subsystem1 : Subsystem
  a : PMIOPort  Side=Right
  b : PMIOPort  Port=2  Side=Right
  c : PMIOPort  Port=3  Side=Right
  A : PMIOPort  Port=4  Side=Left
  B : PMIOPort  Port=5  Side=Left
  C : PMIOPort  Port=6  Side=Left
  Med_n2 : Outport
  wires:
  Subsystem/1(Vabc) -> [Vabc]
  Subsystem1/1(i) -> [Iabc]
  [Vabc] -> Mux/1
  [Iabc] -> Mux/2
  Mux/1 -> Med_n2/1
  connections:
  Subsystem/LConn2 -- Subsystem1/RConn2 -- B/RConn1
  Subsystem1/RConn1 -- Subsystem/LConn1 -- A/RConn1
  Subsystem/LConn3 -- Subsystem1/RConn3 -- C/RConn1
  c/RConn1 -- Subsystem1/LConn3
  Subsystem1/LConn2 -- b/RConn1
  a/RConn1 -- Subsystem1/LConn1

== system HOYAS_GRANDES_I/SM_Computation/HOYAS GRANDES CT01/HG.1_CT.1-INV.07 ==
  Mux : Mux  Inputs=2
  Subsystem : Subsystem
  Subsystem1 : Subsystem
  a : PMIOPort  Side=Right
  b : PMIOPort  Port=2  Side=Right
  c : PMIOPort  Port=3  Side=Right
  A : PMIOPort  Port=4  Side=Left
  B : PMIOPort  Port=5  Side=Left
  C : PMIOPort  Port=6  Side=Left
  Med_n2 : Outport
  wires:
  Mux/1 -> Med_n2/1
  [Iabc] -> Mux/2
  [Vabc] -> Mux/1
  Subsystem1/1(i) -> [Iabc]
  Subsystem/1(Vabc) -> [Vabc]
  connections:
  a/RConn1 -- Subsystem1/LConn1
  Subsystem1/LConn2 -- b/RConn1
  c/RConn1 -- Subsystem1/LConn3
  C/RConn1 -- Subsystem1/RConn3 -- Subsystem/LConn3
  A/RConn1 -- Subsystem/LConn1 -- Subsystem1/RConn1
  B/RConn1 -- Subsystem1/RConn2 -- Subsystem/LConn2

== system HOYAS_GRANDES_I/SM_Computation/HOYAS GRANDES CT01/HG.1_CT.1-INV.08 ==
  Mux : Mux  Inputs=2
  Subsystem : Subsystem
  Subsystem1 : Subsystem
  a : PMIOPort  Side=Right
  b : PMIOPort  Port=2  Side=Right
  c : PMIOPort  Port=3  Side=Right
  A : PMIOPort  Port=4  Side=Left
  B : PMIOPort  Port=5  Side=Left
  C : PMIOPort  Port=6  Side=Left
  Med_n2 : Outport
  wires:
  Subsystem/1(Vabc) -> [Vabc]
  Subsystem1/1(i) -> [Iabc]
  [Vabc] -> Mux/1
  [Iabc] -> Mux/2
  Mux/1 -> Med_n2/1
  connections:
  Subsystem/LConn2 -- Subsystem1/RConn2 -- B/RConn1
  Subsystem1/RConn1 -- Subsystem/LConn1 -- A/RConn1
  Subsystem/LConn3 -- Subsystem1/RConn3 -- C/RConn1
  c/RConn1 -- Subsystem1/LConn3
  Subsystem1/LConn2 -- b/RConn1
  a/RConn1 -- Subsystem1/LConn1

== system HOYAS_GRANDES_I/SM_Computation/HOYAS GRANDES CT01/HG.1_CT.1-INV.09 ==
  Mux : Mux  Inputs=2
  Subsystem : Subsystem
  Subsystem1 : Subsystem
  a : PMIOPort  Side=Right
  b : PMIOPort  Port=2  Side=Right
  c : PMIOPort  Port=3  Side=Right
  A : PMIOPort  Port=4  Side=Left
  B : PMIOPort  Port=5  Side=Left
  C : PMIOPort  Port=6  Side=Left
  Med_n2 : Outport
  wires:
  Mux/1 -> Med_n2/1
  [Iabc] -> Mux/2
  [Vabc] -> Mux/1
  Subsystem1/1(i) -> [Iabc]
  Subsystem/1(Vabc) -> [Vabc]
  connections:
  a/RConn1 -- Subsystem1/LConn1
  Subsystem1/LConn2 -- b/RConn1
  c/RConn1 -- Subsystem1/LConn3
  C/RConn1 -- Subsystem1/RConn3 -- Subsystem/LConn3
  A/RConn1 -- Subsystem/LConn1 -- Subsystem1/RConn1
  B/RConn1 -- Subsystem1/RConn2 -- Subsystem/LConn2

== system HOYAS_GRANDES_I/SM_Computation/HOYAS GRANDES CT01/HG.1_CT.1-INV.10 ==
  Mux : Mux  Inputs=2
  Subsystem : Subsystem
  Subsystem1 : Subsystem
  a : PMIOPort  Side=Right
  b : PMIOPort  Port=2  Side=Right
  c : PMIOPort  Port=3  Side=Right
  A : PMIOPort  Port=4  Side=Left
  B : PMIOPort  Port=5  Side=Left
  C : PMIOPort  Port=6  Side=Left
  Med_n2 : Outport
  wires:
  Subsystem/1(Vabc) -> [Vabc]
  Subsystem1/1(i) -> [Iabc]
  [Vabc] -> Mux/1
  [Iabc] -> Mux/2
  Mux/1 -> Med_n2/1
  connections:
  Subsystem/LConn2 -- Subsystem1/RConn2 -- B/RConn1
  Subsystem1/RConn1 -- Subsystem/LConn1 -- A/RConn1
  Subsystem/LConn3 -- Subsystem1/RConn3 -- C/RConn1
  c/RConn1 -- Subsystem1/LConn3
  Subsystem1/LConn2 -- b/RConn1
  a/RConn1 -- Subsystem1/LConn1

== system HOYAS_GRANDES_I/SM_Computation/HOYAS GRANDES CT01/Medidor18 ==
  Mux : Mux  Inputs=2
  Subsystem : Subsystem
  Subsystem1 : Subsystem
  a : PMIOPort  Side=Right
  b : PMIOPort  Port=2  Side=Right
  c : PMIOPort  Port=3  Side=Right
  A : PMIOPort  Port=4  Side=Left
  B : PMIOPort  Port=5  Side=Left
  C : PMIOPort  Port=6  Side=Left
  Med_n2 : Outport
  wires:
  Mux/1 -> Med_n2/1
  [Iabc] -> Mux/2
  [Vabc] -> Mux/1
  Subsystem1/1(i) -> [Iabc]
  Subsystem/1(Vabc) -> [Vabc]
  connections:
  a/RConn1 -- Subsystem1/LConn1
  Subsystem1/LConn2 -- b/RConn1
  c/RConn1 -- Subsystem1/LConn3
  C/RConn1 -- Subsystem1/RConn3 -- Subsystem/LConn3
  A/RConn1 -- Subsystem/LConn1 -- Subsystem1/RConn1
  B/RConn1 -- Subsystem1/RConn2 -- Subsystem/LConn2

== system HOYAS_GRANDES_I/SM_Computation/HOYAS GRANDES CT02/HG.1-CT.2-INV.01 ==
  PQ : Inport
  Three-Phase Dynamic Load : spsThreePhaseDynamicLoadLib/Three-Phase Dynamic Load  NominalVoltage=[ 800 50 ]  ActiveReactivePowers=[0 0]  PositiveSequence=[1 0]  ExternalControl=on  NpNq=[1.3 2]  TimeConstants="[0  0  0  0]"  MinimumVoltage=0.7  Tfilter=1e-4  LoadFlowParameters=[4,0,0,0,0]
      settings: LibrarySourceBlock=|
      | sps_lib/Passives/Three-Phase
      | Dynamic Load
  Three-Phase Series RLC Branch10 : spsThreePhaseSeriesRLCBranchLib/Three-Phase Series RLC Branch  LConnTagsString=A|B|C  RConnTagsString=A|B|C  BranchType=R  Resistance=1e6  Inductance=X_ac*L  Capacitance=1e-6  Measurements=None
  A : PMIOPort  Side=Right
  B : PMIOPort  Port=2  Side=Right
  C : PMIOPort  Port=3  Side=Right
  m : Outport
  wires:
  PQ/1 -> Three-Phase Dynamic Load/1
  Three-Phase Dynamic Load/1 -> m/1
  connections:
  A/RConn1 -- Three-Phase Dynamic Load/LConn1 -- Three-Phase Series RLC Branch10/RConn1
  Three-Phase Series RLC Branch10/LConn2 -- Three-Phase Series RLC Branch10/LConn3 -- Three-Phase Series RLC Branch10/LConn1
  B/RConn1 -- Three-Phase Series RLC Branch10/RConn2 -- Three-Phase Dynamic Load/LConn2
  Three-Phase Series RLC Branch10/RConn3 -- C/RConn1 -- Three-Phase Dynamic Load/LConn3

== system HOYAS_GRANDES_I/SM_Computation/HOYAS GRANDES CT02/HG.1-CT.2-INV.02 ==
  PQ : Inport
  Three-Phase Dynamic Load : spsThreePhaseDynamicLoadLib/Three-Phase Dynamic Load  NominalVoltage=[ 800 50 ]  ActiveReactivePowers=[0 0]  PositiveSequence=[1 0]  ExternalControl=on  NpNq=[1.3 2]  TimeConstants="[0  0  0  0]"  MinimumVoltage=0.7  Tfilter=1e-4  LoadFlowParameters=[4,0,0,0,0]
      settings: LibrarySourceBlock=|
      | sps_lib/Passives/Three-Phase
      | Dynamic Load
  Three-Phase Series RLC Branch10 : spsThreePhaseSeriesRLCBranchLib/Three-Phase Series RLC Branch  LConnTagsString=A|B|C  RConnTagsString=A|B|C  BranchType=R  Resistance=1e6  Inductance=X_ac*L  Capacitance=1e-6  Measurements=None
  A : PMIOPort  Side=Right
  B : PMIOPort  Port=2  Side=Right
  C : PMIOPort  Port=3  Side=Right
  m : Outport
  wires:
  Three-Phase Dynamic Load/1 -> m/1
  PQ/1 -> Three-Phase Dynamic Load/1
  connections:
  Three-Phase Series RLC Branch10/RConn3 -- Three-Phase Dynamic Load/LConn3 -- C/RConn1
  Three-Phase Dynamic Load/LConn2 -- Three-Phase Series RLC Branch10/RConn2 -- B/RConn1
  Three-Phase Series RLC Branch10/LConn2 -- Three-Phase Series RLC Branch10/LConn1 -- Three-Phase Series RLC Branch10/LConn3
  A/RConn1 -- Three-Phase Series RLC Branch10/RConn1 -- Three-Phase Dynamic Load/LConn1

== system HOYAS_GRANDES_I/SM_Computation/HOYAS GRANDES CT02/HG.1-CT.2-INV.03 ==
  PQ : Inport
  Three-Phase Dynamic Load : spsThreePhaseDynamicLoadLib/Three-Phase Dynamic Load  NominalVoltage=[ 800 50 ]  ActiveReactivePowers=[0 0]  PositiveSequence=[1 0]  ExternalControl=on  NpNq=[1.3 2]  TimeConstants="[0  0  0  0]"  MinimumVoltage=0.7  Tfilter=1e-4  LoadFlowParameters=[4,0,0,0,0]
      settings: LibrarySourceBlock=|
      | sps_lib/Passives/Three-Phase
      | Dynamic Load
  Three-Phase Series RLC Branch10 : spsThreePhaseSeriesRLCBranchLib/Three-Phase Series RLC Branch  LConnTagsString=A|B|C  RConnTagsString=A|B|C  BranchType=R  Resistance=1e6  Inductance=X_ac*L  Capacitance=1e-6  Measurements=None
  A : PMIOPort  Side=Right
  B : PMIOPort  Port=2  Side=Right
  C : PMIOPort  Port=3  Side=Right
  m : Outport
  wires:
  PQ/1 -> Three-Phase Dynamic Load/1
  Three-Phase Dynamic Load/1 -> m/1
  connections:
  Three-Phase Dynamic Load/LConn1 -- Three-Phase Series RLC Branch10/RConn1 -- A/RConn1
  Three-Phase Series RLC Branch10/LConn3 -- Three-Phase Series RLC Branch10/LConn1 -- Three-Phase Series RLC Branch10/LConn2
  B/RConn1 -- Three-Phase Series RLC Branch10/RConn2 -- Three-Phase Dynamic Load/LConn2
  C/RConn1 -- Three-Phase Dynamic Load/LConn3 -- Three-Phase Series RLC Branch10/RConn3

== system HOYAS_GRANDES_I/SM_Computation/HOYAS GRANDES CT02/HG.1-CT.2-INV.04 ==
  PQ : Inport
  Three-Phase Dynamic Load : spsThreePhaseDynamicLoadLib/Three-Phase Dynamic Load  NominalVoltage=[ 800 50 ]  ActiveReactivePowers=[0 0]  PositiveSequence=[1 0]  ExternalControl=on  NpNq=[1.3 2]  TimeConstants="[0  0  0  0]"  MinimumVoltage=0.7  Tfilter=1e-4  LoadFlowParameters=[4,0,0,0,0]
      settings: LibrarySourceBlock=|
      | sps_lib/Passives/Three-Phase
      | Dynamic Load
  Three-Phase Series RLC Branch10 : spsThreePhaseSeriesRLCBranchLib/Three-Phase Series RLC Branch  LConnTagsString=A|B|C  RConnTagsString=A|B|C  BranchType=R  Resistance=1e6  Inductance=X_ac*L  Capacitance=1e-6  Measurements=None
  A : PMIOPort  Side=Right
  B : PMIOPort  Port=2  Side=Right
  C : PMIOPort  Port=3  Side=Right
  m : Outport
  wires:
  Three-Phase Dynamic Load/1 -> m/1
  PQ/1 -> Three-Phase Dynamic Load/1
  connections:
  Three-Phase Series RLC Branch10/RConn3 -- Three-Phase Dynamic Load/LConn3 -- C/RConn1
  Three-Phase Dynamic Load/LConn2 -- Three-Phase Series RLC Branch10/RConn2 -- B/RConn1
  Three-Phase Series RLC Branch10/LConn2 -- Three-Phase Series RLC Branch10/LConn1 -- Three-Phase Series RLC Branch10/LConn3
  A/RConn1 -- Three-Phase Series RLC Branch10/RConn1 -- Three-Phase Dynamic Load/LConn1

== system HOYAS_GRANDES_I/SM_Computation/HOYAS GRANDES CT02/HG.1-CT.2-INV.05 ==
  PQ : Inport
  Three-Phase Dynamic Load : spsThreePhaseDynamicLoadLib/Three-Phase Dynamic Load  NominalVoltage=[ 800 50 ]  ActiveReactivePowers=[0 0]  PositiveSequence=[1 0]  ExternalControl=on  NpNq=[1.3 2]  TimeConstants="[0  0  0  0]"  MinimumVoltage=0.7  Tfilter=1e-4  LoadFlowParameters=[4,0,0,0,0]
      settings: LibrarySourceBlock=|
      | sps_lib/Passives/Three-Phase
      | Dynamic Load
  Three-Phase Series RLC Branch10 : spsThreePhaseSeriesRLCBranchLib/Three-Phase Series RLC Branch  LConnTagsString=A|B|C  RConnTagsString=A|B|C  BranchType=R  Resistance=1e6  Inductance=X_ac*L  Capacitance=1e-6  Measurements=None
  A : PMIOPort  Side=Right
  B : PMIOPort  Port=2  Side=Right
  C : PMIOPort  Port=3  Side=Right
  m : Outport
  wires:
  PQ/1 -> Three-Phase Dynamic Load/1
  Three-Phase Dynamic Load/1 -> m/1
  connections:
  Three-Phase Dynamic Load/LConn1 -- Three-Phase Series RLC Branch10/RConn1 -- A/RConn1
  Three-Phase Series RLC Branch10/LConn3 -- Three-Phase Series RLC Branch10/LConn1 -- Three-Phase Series RLC Branch10/LConn2
  B/RConn1 -- Three-Phase Series RLC Branch10/RConn2 -- Three-Phase Dynamic Load/LConn2
  C/RConn1 -- Three-Phase Dynamic Load/LConn3 -- Three-Phase Series RLC Branch10/RConn3

== system HOYAS_GRANDES_I/SM_Computation/HOYAS GRANDES CT02/HG.1-CT.2-INV.06 ==
  PQ : Inport
  Three-Phase Dynamic Load : spsThreePhaseDynamicLoadLib/Three-Phase Dynamic Load  NominalVoltage=[ 800 50 ]  ActiveReactivePowers=[0 0]  PositiveSequence=[1 0]  ExternalControl=on  NpNq=[1.3 2]  TimeConstants="[0  0  0  0]"  MinimumVoltage=0.7  Tfilter=1e-4  LoadFlowParameters=[4,0,0,0,0]
      settings: LibrarySourceBlock=|
      | sps_lib/Passives/Three-Phase
      | Dynamic Load
  Three-Phase Series RLC Branch10 : spsThreePhaseSeriesRLCBranchLib/Three-Phase Series RLC Branch  LConnTagsString=A|B|C  RConnTagsString=A|B|C  BranchType=R  Resistance=1e6  Inductance=X_ac*L  Capacitance=1e-6  Measurements=None
  A : PMIOPort  Side=Right
  B : PMIOPort  Port=2  Side=Right
  C : PMIOPort  Port=3  Side=Right
  m : Outport
  wires:
  Three-Phase Dynamic Load/1 -> m/1
  PQ/1 -> Three-Phase Dynamic Load/1
  connections:
  Three-Phase Series RLC Branch10/RConn3 -- Three-Phase Dynamic Load/LConn3 -- C/RConn1
  Three-Phase Dynamic Load/LConn2 -- Three-Phase Series RLC Branch10/RConn2 -- B/RConn1
  Three-Phase Series RLC Branch10/LConn2 -- Three-Phase Series RLC Branch10/LConn1 -- Three-Phase Series RLC Branch10/LConn3
  A/RConn1 -- Three-Phase Series RLC Branch10/RConn1 -- Three-Phase Dynamic Load/LConn1

== system HOYAS_GRANDES_I/SM_Computation/HOYAS GRANDES CT02/HG.1-CT.2-INV.07 ==
  PQ : Inport
  Three-Phase Dynamic Load : spsThreePhaseDynamicLoadLib/Three-Phase Dynamic Load  NominalVoltage=[ 800 50 ]  ActiveReactivePowers=[0 0]  PositiveSequence=[1 0]  ExternalControl=on  NpNq=[1.3 2]  TimeConstants="[0  0  0  0]"  MinimumVoltage=0.7  Tfilter=1e-4  LoadFlowParameters=[4,0,0,0,0]
      settings: LibrarySourceBlock=|
      | sps_lib/Passives/Three-Phase
      | Dynamic Load
  Three-Phase Series RLC Branch10 : spsThreePhaseSeriesRLCBranchLib/Three-Phase Series RLC Branch  LConnTagsString=A|B|C  RConnTagsString=A|B|C  BranchType=R  Resistance=1e6  Inductance=X_ac*L  Capacitance=1e-6  Measurements=None
  A : PMIOPort  Side=Right
  B : PMIOPort  Port=2  Side=Right
  C : PMIOPort  Port=3  Side=Right
  m : Outport
  wires:
  PQ/1 -> Three-Phase Dynamic Load/1
  Three-Phase Dynamic Load/1 -> m/1
  connections:
  Three-Phase Dynamic Load/LConn1 -- Three-Phase Series RLC Branch10/RConn1 -- A/RConn1
  Three-Phase Series RLC Branch10/LConn3 -- Three-Phase Series RLC Branch10/LConn1 -- Three-Phase Series RLC Branch10/LConn2
  B/RConn1 -- Three-Phase Series RLC Branch10/RConn2 -- Three-Phase Dynamic Load/LConn2
  C/RConn1 -- Three-Phase Dynamic Load/LConn3 -- Three-Phase Series RLC Branch10/RConn3

== system HOYAS_GRANDES_I/SM_Computation/HOYAS GRANDES CT02/HG.1-CT.2-INV.08 ==
  PQ : Inport
  Three-Phase Dynamic Load : spsThreePhaseDynamicLoadLib/Three-Phase Dynamic Load  NominalVoltage=[ 800 50 ]  ActiveReactivePowers=[0 0]  PositiveSequence=[1 0]  ExternalControl=on  NpNq=[1.3 2]  TimeConstants="[0  0  0  0]"  MinimumVoltage=0.7  Tfilter=1e-4  LoadFlowParameters=[4,0,0,0,0]
      settings: LibrarySourceBlock=|
      | sps_lib/Passives/Three-Phase
      | Dynamic Load
  Three-Phase Series RLC Branch10 : spsThreePhaseSeriesRLCBranchLib/Three-Phase Series RLC Branch  LConnTagsString=A|B|C  RConnTagsString=A|B|C  BranchType=R  Resistance=1e6  Inductance=X_ac*L  Capacitance=1e-6  Measurements=None
  A : PMIOPort  Side=Right
  B : PMIOPort  Port=2  Side=Right
  C : PMIOPort  Port=3  Side=Right
  m : Outport
  wires:
  Three-Phase Dynamic Load/1 -> m/1
  PQ/1 -> Three-Phase Dynamic Load/1
  connections:
  Three-Phase Series RLC Branch10/RConn3 -- Three-Phase Dynamic Load/LConn3 -- C/RConn1
  Three-Phase Dynamic Load/LConn2 -- Three-Phase Series RLC Branch10/RConn2 -- B/RConn1
  Three-Phase Series RLC Branch10/LConn2 -- Three-Phase Series RLC Branch10/LConn1 -- Three-Phase Series RLC Branch10/LConn3
  A/RConn1 -- Three-Phase Series RLC Branch10/RConn1 -- Three-Phase Dynamic Load/LConn1
